simulink model "Elicottero2DOF_Sim"  (R2026a)
settings: Solver=VariableStepAuto  StopTime=20  FixedStep=0.0005
values from neighbouring files (symbols this model uses):
  M_0 = 46.5    [Elicottero2DOF_INIT.m]
  m_treshold = 3    [Elicottero2DOF_INIT.m]
  MAHALANOBIS = false    [Elicottero2DOF_INIT.m]
  Outlier_flag = 0    [Elicottero2DOF_INIT.m]
  P0 = diag([P_0_alpha P_0_alpha_dot P_0_beta P_0_beta_dot])    [Elicottero2DOF_INIT.m]
  q_0 = [alpha_0 beta_0]'    [Elicottero2DOF_INIT.m]
  q_dot_0 = [alpha_dot_0 beta_dot_0]'    [Elicottero2DOF_INIT.m]
  seme_rumore = 12345    [Elicottero2DOF_INIT.m]
  sigma_acc = 0.0137    [Elicottero2DOF_INIT.m]
  sigma_magn = 0.14    [Elicottero2DOF_INIT.m]
  st_acc = 0.00435    [Elicottero2DOF_INIT.m]
  st_magn = 0.005    [Elicottero2DOF_INIT.m]
  x_0 = [(deg2rad(10) + deg2rad(3)) 0.05 deg2rad(5) -0.05]'    [Elicottero2DOF_INIT.m]
undefined symbols (not defined in the file or in its folder): params
libraries: simulink x2
settings Model: Creator=giggi  LastModifiedBy=giggi

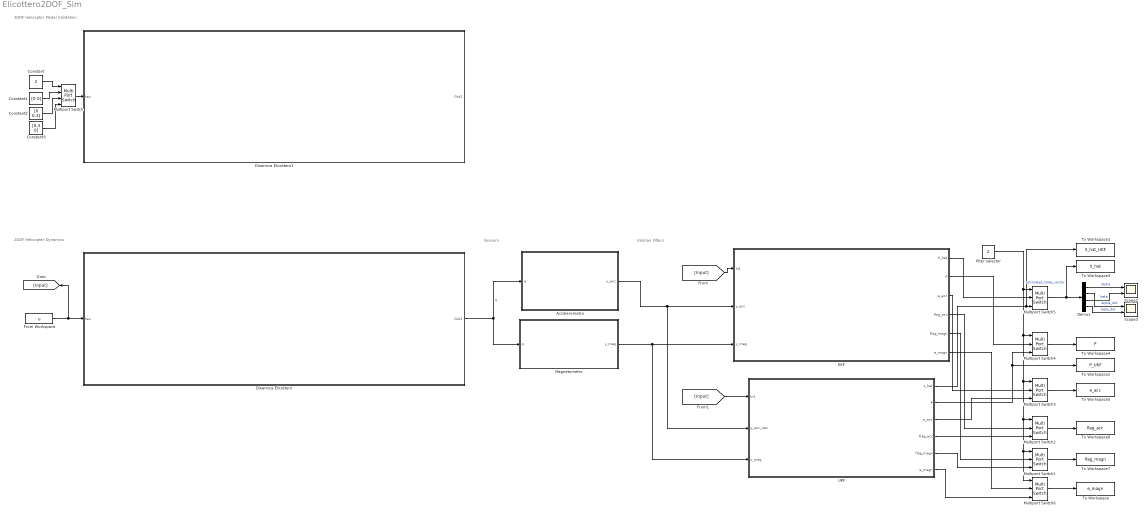
== system Elicottero2DOF_Sim ==
  note: Kalman FIlters
  note: 2DOF Helicopter Dynamics
  note: Sensors
  note: 2DOF Helicopter Model Validation
  Accelerometro : Subsystem
  Constant : Constant  Value=2
  Constant1 : Constant  Value=[0 0]
  Constant2 : Constant  Value=[0 0.3]
  Constant3 : Constant  Value=[0.3 0]
  Demux : Demux
  Dinamica Elicottero : Subsystem
  Dinamica Elicottero1 : Subsystem
  EKF : Subsystem
  From Workspace : FromWorkspace  VariableName=u  SampleTime=params.st
  Magnetometro : Subsystem
  Multiport Switch : MultiPortSwitch  SaturateOnIntegerOverflow=off  InputSameDT=off
  Multiport Switch{1..6} (6 alike) : MultiPortSwitch  Inputs=2  SaturateOnIntegerOverflow=off  InputSameDT=off
  Scope2 : Scope  NumInputPorts=2
      settings: ActiveDisplayYMinimum=-0.071075894197221115  ActiveDisplayYMaximum=0.60556663596837657  DataLoggingVariableName=ScopeData7
  Scope3 : Scope  NumInputPorts=2
      settings: ActiveDisplayYMinimum=-0.27957788580280007  ActiveDisplayYMaximum=0.23844227860003075  DataLoggingVariableName=ScopeData11
  To Workspace : ToWorkspace  VariableName=e_magn  SaveFormat=Timeseries  SampleTime=params.st
  To Workspace1 : ToWorkspace  VariableName=X_hat_UKF  SaveFormat=Timeseries  SampleTime=params.st
  To Workspace2 : ToWorkspace  VariableName=P_UKF  SaveFormat=Timeseries  SampleTime=params.st
  To Workspace3 : ToWorkspace  VariableName=X_hat  SaveFormat=Timeseries  SampleTime=params.st
  To Workspace4 : ToWorkspace  VariableName=P  SaveFormat=Timeseries  SampleTime=params.st
  To Workspace5 : ToWorkspace  VariableName=e_acc  SaveFormat=Timeseries  SampleTime=params.st
  To Workspace6 : ToWorkspace  VariableName=flag_acc  SaveFormat=Timeseries  SampleTime=params.st
  To Workspace7 : ToWorkspace  VariableName=flag_magn  SaveFormat=Timeseries  SampleTime=params.st
  UKF : Subsystem
  filter selector : Constant  Value=2
  wires:
  From Workspace/1 -> Dinamica Elicottero/1(tau), [Input]
  Dinamica Elicottero/1(Out1) -> Magnetometro/1(q), Accelerometro/1(q)  "q"
  [Input] -> EKF/1(In1)
  [Input] -> UKF/1(In1)
  Accelerometro/1(y_acc) -> UKF/2(y_acc_raw), EKF/2(y_acc)
  Magnetometro/1(y_mag) -> UKF/3(y_mag), EKF/3(y_mag)
  Constant/1 -> Multiport Switch/1
  Constant1/1 -> Multiport Switch/2
  Constant2/1 -> Multiport Switch/3
  Constant3/1 -> Multiport Switch/4
  Multiport Switch/1 -> Dinamica Elicottero1/1(tau)
  Demux/4 -> Scope3/2  "beta_dot"
  Demux/1 -> Scope2/1  "alpha"
  Demux/3 -> Scope2/2  "beta"
  Multiport Switch4/1 -> To Workspace4/1
  Demux/2 -> Scope3/1  "alpha_dot"
  Multiport Switch1/1 -> To Workspace7/1
  UKF/5(flag_magn) -> Multiport Switch1/3
  UKF/4(flag_acc) -> Multiport Switch2/3
  Multiport Switch2/1 -> To Workspace6/1
  UKF/3(e_acc) -> Multiport Switch3/3
  Multiport Switch3/1 -> To Workspace5/1
  Multiport Switch5/1 -> Demux/1, To Workspace3/1  "estimated_state_vector"
  UKF/2(P) -> Multiport Switch4/3, To Workspace2/1
  EKF/1(X_hat) -> Multiport Switch5/2
  UKF/1(x_hat) -> Multiport Switch5/3, To Workspace1/1
  EKF/2(P) -> Multiport Switch4/2
  EKF/3(e_acc) -> Multiport Switch3/2
  EKF/4(flag_acc) -> Multiport Switch2/2
  EKF/5(flag_magn) -> Multiport Switch1/2
  filter selector/1 -> Multiport Switch6/1, Multiport Switch1/1, Multiport Switch2/1, Multiport Switch3/1, Multiport Switch4/1, Multiport Switch5/1
  Multiport Switch6/1 -> To Workspace/1
  EKF/6(e_magn) -> Multiport Switch6/2
  UKF/6(e_magn) -> Multiport Switch6/3

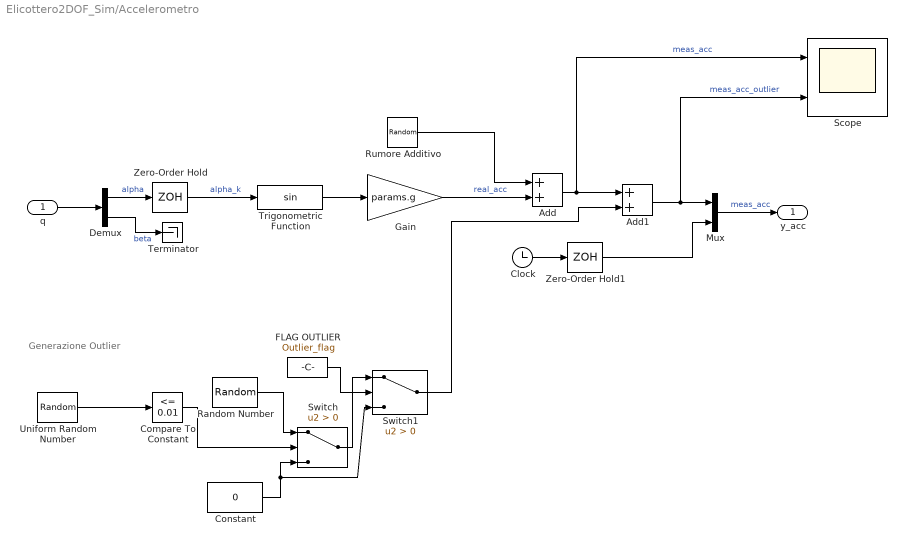
== system Elicottero2DOF_Sim/Accelerometro ==
  note: Generazione Outlier
  q : Inport
  Add : Sum
  Add1 : Sum
  Clock : Clock
  Compare To Constant : simulink/Logic and Bit Operations/Compare To Constant  relop=<=  const=0.01  OutDataTypeStr=boolean
  Constant : Constant  Value=0  SampleTime=st_acc
  Demux : Demux  Outputs=2
  FLAG OUTLIER : Constant  Value=Outlier_flag  SampleTime=st_acc
  Gain : Gain  Gain=params.g
  Mux : Mux  Inputs=2
  Random Number : RandomNumber  Variance=100  Seed=seme_rumore + 18  SampleTime=st_acc
  Rumore Additivo : RandomNumber  Variance=sigma_acc^2  Seed=seme_rumore  SampleTime=st_acc
  Scope : Scope  NumInputPorts=2
      settings: ActiveDisplayYMinimum=-1.7650304215432193  ActiveDisplayYMaximum=2.1182246618135347
  Switch : Switch  Criteria=u2 > Threshold  SaturateOnIntegerOverflow=off  InputSameDT=off
  Switch1 : Switch  Criteria=u2 > Threshold  SaturateOnIntegerOverflow=off  InputSameDT=off
  Terminator : Terminator
  Trigonometric Function : Trigonometry
  Uniform Random Number : UniformRandomNumber  Minimum=0  Seed=seme_rumore + 953  SampleTime=st_acc
  Zero-Order Hold : ZeroOrderHold  SampleTime=st_acc
  Zero-Order Hold1 : ZeroOrderHold  SampleTime=st_acc
  y_acc : Outport
  wires:
  q/1 -> Demux/1
  Demux/1 -> Zero-Order Hold/1  "alpha"
  Demux/2 -> Terminator/1  "beta"
  Trigonometric Function/1 -> Gain/1
  Gain/1 -> Add/2  "real_acc"
  Rumore Additivo/1 -> Add/1
  Add/1 -> Scope/1, Add1/1  "meas_acc"
  Zero-Order Hold/1 -> Trigonometric Function/1  "alpha_k"
  Mux/1 -> y_acc/1  "meas_acc"
  Clock/1 -> Zero-Order Hold1/1
  Zero-Order Hold1/1 -> Mux/2
  FLAG OUTLIER/1 -> Switch1/2
  Constant/1 -> Switch1/3, Switch/3
  Compare To Constant/1 -> Switch/2
  Random Number/1 -> Switch/1
  Switch/1 -> Switch1/1
  Switch1/1 -> Add1/2
  Uniform Random Number/1 -> Compare To Constant/1
  Add1/1 -> Scope/2, Mux/1  "meas_acc_outlier"

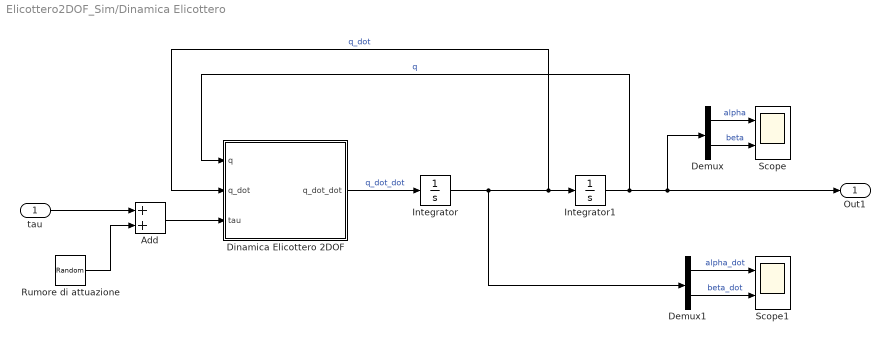
== system Elicottero2DOF_Sim/Dinamica Elicottero ==
  tau : Inport
  Add : Sum
  Demux : Demux  Outputs=2
  Demux1 : Demux  Outputs=2
  Dinamica Elicottero 2DOF : MATLAB Function  TreatAsAtomicUnit=on
  Integrator : Integrator  InitialCondition=q_dot_0
  Integrator1 : Integrator  InitialCondition=q_0
  Rumore di attuazione : RandomNumber  Mean=[0 0]  Variance=[params.sigma_F params.sigma_F].^2  Seed=seme_rumore + 15  SampleTime=params.st
  Scope : Scope  NumInputPorts=2
      settings: ActiveDisplayYMinimum=-0.1777950485917946  ActiveDisplayYMaximum=0.21368047784290267
  Scope1 : Scope  NumInputPorts=2
      settings: ActiveDisplayYMinimum=-0.28050979862132908  ActiveDisplayYMaximum=0.27285629021011787  DataLoggingVariableName=ScopeData4
  Out1 : Outport
  wires:
  Demux/1 -> Scope/1  "alpha"
  Integrator1/1 -> Out1/1, Demux/1, Dinamica Elicottero 2DOF/1(q)  "q"
  Dinamica Elicottero 2DOF/1(q_dot_dot) -> Integrator/1  "q_dot_dot"
  Demux/2 -> Scope/2  "beta"
  Demux1/1 -> Scope1/1  "alpha_dot"
  Demux1/2 -> Scope1/2  "beta_dot"
  Integrator/1 -> Demux1/1, Dinamica Elicottero 2DOF/2(q_dot), Integrator1/1  "q_dot"
  tau/1 -> Add/1
  Add/1 -> Dinamica Elicottero 2DOF/3(tau)
  Rumore di attuazione/1 -> Add/2

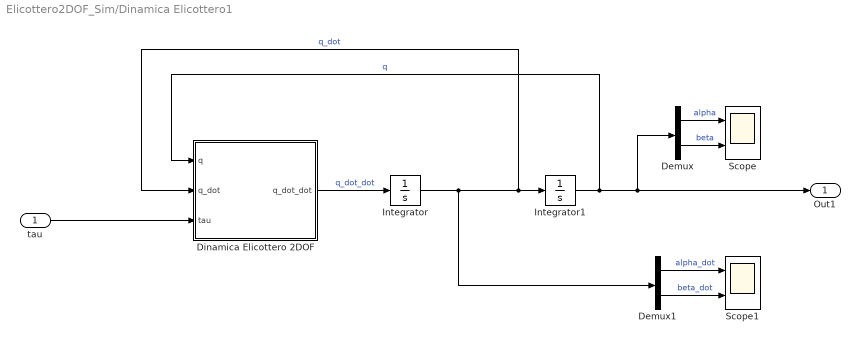
== system Elicottero2DOF_Sim/Dinamica Elicottero1 ==
  tau : Inport
  Demux : Demux  Outputs=2
  Demux1 : Demux  Outputs=2
  Dinamica Elicottero 2DOF : MATLAB Function  TreatAsAtomicUnit=on
  Integrator : Integrator  InitialCondition=q_dot_0
  Integrator1 : Integrator  InitialCondition=q_0
  Scope : Scope  NumInputPorts=2
      settings: ActiveDisplayYMinimum=-14.088875046539977  ActiveDisplayYMaximum=126.79987541885983
  Scope1 : Scope  NumInputPorts=2
      settings: ActiveDisplayYMinimum=-0.74875373653795674  ActiveDisplayYMaximum=6.7387836288416114  DataLoggingVariableName=ScopeData4
  Out1 : Outport
  wires:
  Demux/1 -> Scope/1  "alpha"
  Integrator1/1 -> Out1/1, Demux/1, Dinamica Elicottero 2DOF/1(q)  "q"
  Dinamica Elicottero 2DOF/1(q_dot_dot) -> Integrator/1  "q_dot_dot"
  Demux/2 -> Scope/2  "beta"
  Demux1/1 -> Scope1/1  "alpha_dot"
  Demux1/2 -> Scope1/2  "beta_dot"
  Integrator/1 -> Demux1/1, Dinamica Elicottero 2DOF/2(q_dot), Integrator1/1  "q_dot"
  tau/1 -> Dinamica Elicottero 2DOF/3(tau)

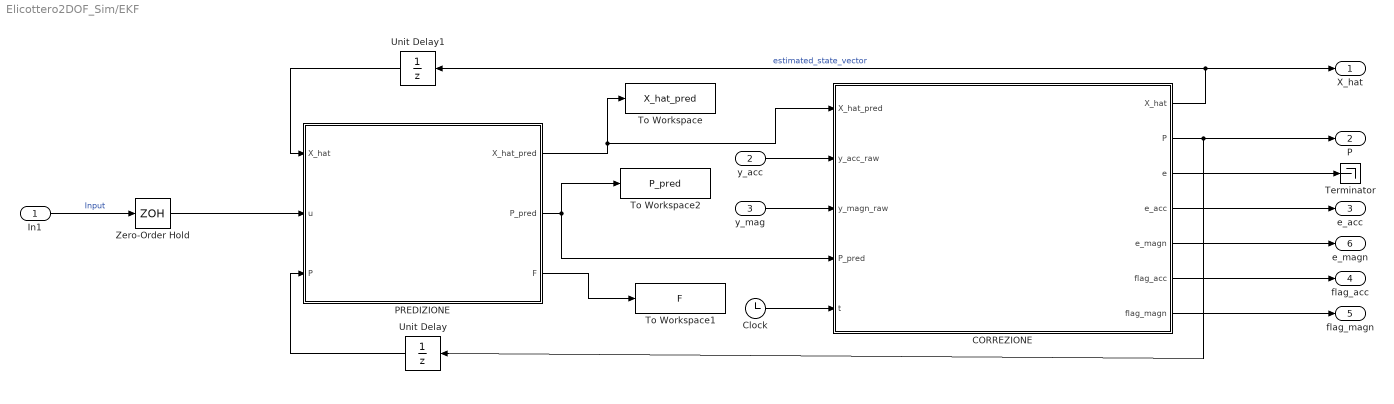
== system Elicottero2DOF_Sim/EKF ==
  In1 : Inport
  y_acc : Inport  Port=2
  y_mag : Inport  Port=3
  CORREZIONE : MATLAB Function  TreatAsAtomicUnit=on
  Clock : Clock
  PREDIZIONE : MATLAB Function  TreatAsAtomicUnit=on
  Terminator : Terminator
  To Workspace : ToWorkspace  VariableName=X_hat_pred  SaveFormat=Timeseries  SampleTime=params.st
  To Workspace1 : ToWorkspace  VariableName=F  SaveFormat=Timeseries  SampleTime=params.st
  To Workspace2 : ToWorkspace  VariableName=P_pred  SaveFormat=Timeseries  SampleTime=params.st
  Unit Delay : UnitDelay  InitialCondition=P0  SampleTime=params.st
  Unit Delay1 : UnitDelay  InitialCondition=x_0  SampleTime=params.st
  Zero-Order Hold : ZeroOrderHold  SampleTime=params.st
  X_hat : Outport
  P : Outport  Port=2
  e_acc : Outport  Port=3
  flag_acc : Outport  Port=4
  flag_magn : Outport  Port=5
  e_magn : Outport  Port=6
  wires:
  PREDIZIONE/2(P_pred) -> To Workspace2/1, CORREZIONE/4(P_pred)
  Zero-Order Hold/1 -> PREDIZIONE/2(u)
  In1/1 -> Zero-Order Hold/1  "Input"
  Unit Delay/1 -> PREDIZIONE/3(P)
  Unit Delay1/1 -> PREDIZIONE/1(X_hat)
  y_acc/1 -> CORREZIONE/2(y_acc_raw)
  y_mag/1 -> CORREZIONE/3(y_magn_raw)
  CORREZIONE/1(X_hat) -> X_hat/1, Unit Delay1/1  "estimated_state_vector"
  PREDIZIONE/1(X_hat_pred) -> To Workspace/1, CORREZIONE/1(X_hat_pred)
  CORREZIONE/2(P) -> Unit Delay/1, P/1
  Clock/1 -> CORREZIONE/5(t)
  PREDIZIONE/3(F) -> To Workspace1/1
  CORREZIONE/4(e_acc) -> e_acc/1
  CORREZIONE/6(flag_acc) -> flag_acc/1
  CORREZIONE/7(flag_magn) -> flag_magn/1
  CORREZIONE/3(e) -> Terminator/1
  CORREZIONE/5(e_magn) -> e_magn/1

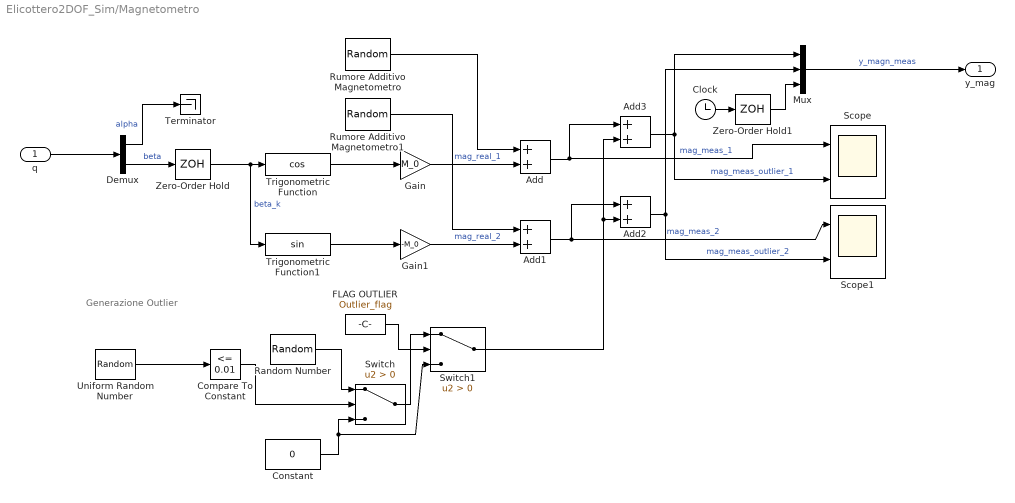
== system Elicottero2DOF_Sim/Magnetometro ==
  note: Generazione Outlier
  q : Inport
  Add{,1..3} (4 alike) : Sum
  Clock : Clock
  Compare To Constant : simulink/Logic and Bit Operations/Compare To Constant  relop=<=  const=0.01  OutDataTypeStr=boolean
  Constant : Constant  Value=0  SampleTime=st_magn
  Demux : Demux  Outputs=2
  FLAG OUTLIER : Constant  Value=Outlier_flag  SampleTime=st_magn
  Gain : Gain  Gain=M_0
  Gain1 : Gain  Gain=-M_0
  Mux : Mux  Inputs=3
  Random Number : RandomNumber  Variance=100  Seed=seme_rumore + 43  SampleTime=st_magn
  Rumore Additivo Magnetometro : RandomNumber  Variance=sigma_magn^2  Seed=seme_rumore + 1  SampleTime=st_magn
  Rumore Additivo Magnetometro1 : RandomNumber  Variance=sigma_magn^2  Seed=seme_rumore + 300  SampleTime=st_magn
  Scope : Scope  NumInputPorts=2
      settings: ActiveDisplayYMinimum=45.876225966404974  ActiveDisplayYMaximum=47.084900080547662  DataLoggingVariableName=ScopeData2
  Scope1 : Scope  NumInputPorts=2
      settings: ActiveDisplayYMinimum=-0.62118665847594379  ActiveDisplayYMaximum=0.61456044976709734  DataLoggingVariableName=ScopeData3
  Switch : Switch  Criteria=u2 > Threshold  SaturateOnIntegerOverflow=off  InputSameDT=off
  Switch1 : Switch  Criteria=u2 > Threshold  SaturateOnIntegerOverflow=off  InputSameDT=off
  Terminator : Terminator
  Trigonometric Function : Trigonometry  Operator=cos
  Trigonometric Function1 : Trigonometry
  Uniform Random Number : UniformRandomNumber  Minimum=0  Seed=seme_rumore + 921  SampleTime=st_magn
  Zero-Order Hold : ZeroOrderHold  SampleTime=st_magn
  Zero-Order Hold1 : ZeroOrderHold  SampleTime=st_magn
  y_mag : Outport
  wires:
  q/1 -> Demux/1
  Demux/2 -> Zero-Order Hold/1  "beta"
  Demux/1 -> Terminator/1  "alpha"
  Trigonometric Function/1 -> Gain/1
  Trigonometric Function1/1 -> Gain1/1
  Gain/1 -> Add/2  "mag_real_1"
  Rumore Additivo Magnetometro/1 -> Add/1
  Gain1/1 -> Add1/2  "mag_real_2"
  Zero-Order Hold/1 -> Trigonometric Function1/1, Trigonometric Function/1  "beta_k"
  Mux/1 -> y_mag/1  "y_magn_meas"
  Clock/1 -> Zero-Order Hold1/1
  Zero-Order Hold1/1 -> Mux/3
  Uniform Random Number/1 -> Compare To Constant/1
  Random Number/1 -> Switch/1
  Compare To Constant/1 -> Switch/2
  Constant/1 -> Switch1/3, Switch/3
  FLAG OUTLIER/1 -> Switch1/2
  Switch/1 -> Switch1/1
  Add/1 -> Scope/1, Add3/1  "mag_meas_1"
  Rumore Additivo Magnetometro1/1 -> Add1/1
  Add2/1 -> Scope1/2, Mux/2  "mag_meas_outlier_2"
  Add1/1 -> Scope1/1, Add2/1  "mag_meas_2"
  Switch1/1 -> Add2/2, Add3/2
  Add3/1 -> Scope/2, Mux/1  "mag_meas_outlier_1"

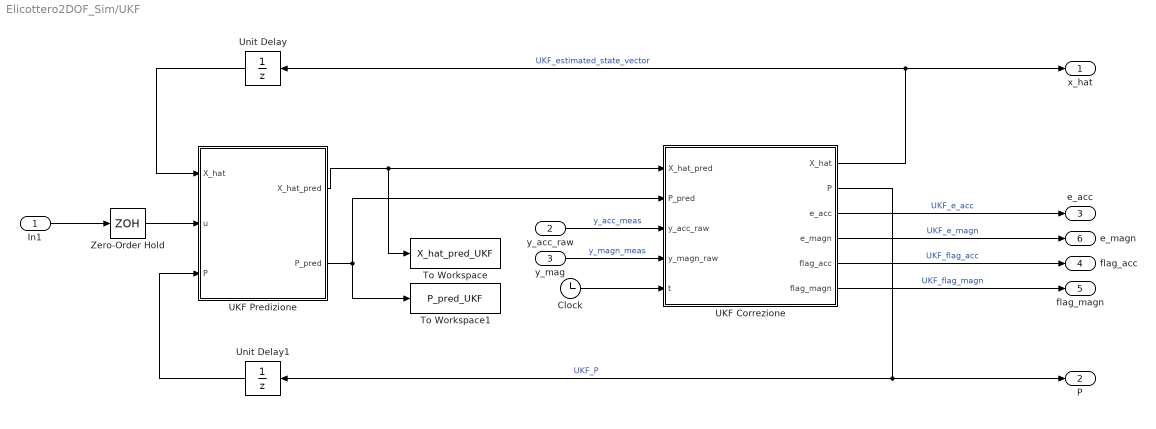
== system Elicottero2DOF_Sim/UKF ==
  In1 : Inport
  y_acc_raw : Inport  Port=2
  y_mag : Inport  Port=3
  Clock : Clock
  To Workspace : ToWorkspace  VariableName=X_hat_pred_UKF  SaveFormat=Timeseries  SampleTime=params.st
  To Workspace1 : ToWorkspace  VariableName=P_pred_UKF  SaveFormat=Timeseries  SampleTime=params.st
  UKF Correzione : MATLAB Function  TreatAsAtomicUnit=on
  UKF Predizione : MATLAB Function  TreatAsAtomicUnit=on
  Unit Delay : UnitDelay  InitialCondition=x_0  SampleTime=params.st
  Unit Delay1 : UnitDelay  InitialCondition=P0  SampleTime=params.st
  Zero-Order Hold : ZeroOrderHold  SampleTime=params.st
  x_hat : Outport
  P : Outport  Port=2
  e_acc : Outport  Port=3
  flag_acc : Outport  Port=4
  flag_magn : Outport  Port=5
  e_magn : Outport  Port=6
  wires:
  Unit Delay/1 -> UKF Predizione/1(X_hat)
  Unit Delay1/1 -> UKF Predizione/3(P)
  In1/1 -> Zero-Order Hold/1
  Zero-Order Hold/1 -> UKF Predizione/2(u)
  y_acc_raw/1 -> UKF Correzione/3(y_acc_raw)  "y_acc_meas"
  y_mag/1 -> UKF Correzione/4(y_magn_raw)  "y_magn_meas"
  UKF Predizione/1(X_hat_pred) -> To Workspace/1, UKF Correzione/1(X_hat_pred)
  UKF Predizione/2(P_pred) -> To Workspace1/1, UKF Correzione/2(P_pred)
  UKF Correzione/1(X_hat) -> x_hat/1, Unit Delay/1  "UKF_estimated_state_vector"
  UKF Correzione/2(P) -> P/1, Unit Delay1/1  "UKF_P"
  UKF Correzione/3(e_acc) -> e_acc/1  "UKF_e_acc"
  Clock/1 -> UKF Correzione/5(t)
  UKF Correzione/6(flag_magn) -> flag_magn/1  "UKF_flag_magn"
  UKF Correzione/5(flag_acc) -> flag_acc/1  "UKF_flag_acc"
  UKF Correzione/4(e_magn) -> e_magn/1  "UKF_e_magn"

== matlab function Elicottero2DOF_Sim/Dinamica Elicottero1/Dinamica Elicottero 2DOF ==
  data: q input; q_dot input; tau input; q_dot_dot output; params parameter
function q_dot_dot = fcn(q, q_dot, tau, params)

alpha = q(1);
alpha_dot = q_dot(1);
beta = q(2);
beta_dot = q_dot(2);

% Costruzione Momento di Inerzia di Yaw (Variabile con angolo di pitch)
J_beta = params.J_y * sin(alpha)^2 + (params.J_z + params.m * params.l^2) * cos(alpha)^2 + params.I_b;

% Matrice di Inerzia
M = [params.J_alpha 0; 0 J_beta];

% Vettore dei termini non lineari (raccoglie attriti viscosi e forza di gravità)
n = [params.c_alpha * alpha_dot + params.m * params.g * params.l * sin(alpha); params.c_beta * beta_dot];

% Vettore delle Forze / Coppie generalizzate
B = [params.l * cos(beta), params.epsilon_p * params.l * sin(beta); params.epsilon_y * params.l * sin(alpha), params.l * cos(alpha)];

% Dinamica Inversa
q_dot_dot = M \ (B * tau - n);

== matlab function Elicottero2DOF_Sim/EKF/PREDIZIONE ==
  data: X_hat input; u input; P input; X_hat_pred output; P_pred output; params parameter; F output
function [X_hat_pred, P_pred, F] = Predizione(X_hat, u, P, params)
    % PREDIZIONE EKF - Modello con Rumore di Attuazione sui Motori
    
    %% 1. Lettura dello Stato e Ingressi
    alpha     = X_hat(1);
    alpha_dot = X_hat(2);
    beta      = X_hat(3);
    beta_dot  = X_hat(4);
    
    F1 = u(1);
    F2 = u(2);
    
    %% 2. Estrazione Parametri Fisici
    m  = params.m;       l  = params.l;       g  = params.g;
    Ja = params.J_alpha; Jy = params.J_y;     Jz = params.J_z;
    Ib = params.I_b;     ca = params.c_alpha; cb = params.c_beta;
    ep = params.epsilon_p;   ey = params.epsilon_y;   
    dt = params.st;
    
    %% 3. Matrice di Covarianza del Rumore di Processo (Q)
    % Q è 2x2. Contiene la varianza del rumore dei motori EMAX MT2204
    % param.sigma_F = 0.05 [Newton]
    Q = [params.sigma_F^2, 0;
         0,               params.sigma_F^2];

    %% 4. MODELLO DINAMICO NON LINEARE
    J_beta = Jy * sin(alpha)^2 + (Jz + m*l^2) * cos(alpha)^2 + Ib;
    
    alpha_ddot = (-ca * alpha_dot - m * g * l * sin(alpha) + ...
                   l * F1 * cos(beta) + ep * l * F2 * sin(beta)) / Ja;
                   
    beta_ddot  = (-cb * beta_dot + l * F2 * cos(alpha) + ...
                   ey * l * F1 * sin(alpha)) / J_beta;

    %% 5. PREDIZIONE DELLO STATO (Eulero)
    X_hat_pred = [alpha     + dt * alpha_dot;
                  alpha_dot + dt * alpha_ddot;
                  beta      + dt * beta_dot;
                  beta_dot  + dt * beta_ddot];

    %% 6. CALCOLO JACOBIANA DI PROCESSO (A) -> F = I + A*dt
    % Derivate per la riga 2 (alpha_ddot)
    A21 = (-m * g * l * cos(alpha)) / Ja;
    A22 = -ca / Ja;
    A23 = (-l * F1 * sin(beta) + ep * l * F2 * cos(beta)) / Ja;
    A24 = 0;
    
    % Derivate per la riga 4 (beta_ddot)
    N = -cb * beta_dot + l * F2 * cos(alpha) + ey * l * F1 * sin(alpha);
    D_den = J_beta;
    dN_dalpha = -l * F2 * sin(alpha) + ey * l * F1 * cos(alpha);
    dD_dalpha = 2 * Jy * sin(alpha) * cos(alpha) - 2 * (Jz + m*l^2) * cos(alpha) * sin(alpha);
    
    A41 = (D_den * dN_dalpha - N * dD_dalpha) / (D_den^2);
    A42 = 0;
    A43 = 0;
    A44 = -cb / D_den;
    
    % Assemblaggio e discretizzazione
    A = [  0,   1,   0,   0;
         A21, A22, A23, A24;
           0,   0,   0,   1;
         A41, A42, A43, A44];
         
    F = eye(4) + A * dt;
    
    %% 7. CALCOLO JACOBIANA DEI DISTURBI (D)
    % Rappresenta l'impatto di 1 Newton di errore del motore sulle accelerazioni.
    % La matrice è 4x2 perché mappa 2 rumori su 4 stati.
    
    d_alpha_ddot_w1 = (l * cos(beta)) / Ja;
    d_alpha_ddot_w2 = (ep * l * sin(beta)) / Ja;
    
    d_beta_ddot_w1  = (ey * l * sin(alpha)) / J_beta;
    d_beta_ddot_w2  = (l * cos(alpha)) / J_beta;
    
    D = [0,                         0;
         d_alpha_ddot_w1 * dt,      d_alpha_ddot_w2 * dt;
         0,                         0;
         d_beta_ddot_w1 * dt,       d_beta_ddot_w2 * dt];
         
    %% 8. PREDIZIONE DELLA COVARIANZA
    % Diffusione dell'incertezza dei motori negli stati tramite la matrice D
    P_pred = F * P * F' + D * Q * D';
    
end

== matlab function Elicottero2DOF_Sim/Dinamica Elicottero/Dinamica Elicottero 2DOF ==
  data: q input; q_dot input; tau input; q_dot_dot output; params parameter
function q_dot_dot = fcn(q, q_dot, tau, params)

alpha = q(1);
alpha_dot = q_dot(1);
beta = q(2);
beta_dot = q_dot(2);

% Costruzione Momento di Inerzia di Yaw (Variabile con angolo di pitch)
J_beta = params.J_y * sin(alpha)^2 + (params.J_z + params.m * params.l^2) * cos(alpha)^2 + params.I_b;

% Matrice di Inerzia
M = [params.J_alpha 0; 0 J_beta];

% Vettore dei termini non lineari (raccoglie attriti viscosi e forza di gravità)
n = [params.c_alpha * alpha_dot + params.m * params.g * params.l * sin(alpha); params.c_beta * beta_dot];

% Vettore delle Forze / Coppie generalizzate
B = [params.l * cos(beta), params.epsilon_p * params.l * sin(beta); params.epsilon_y * params.l * sin(alpha), params.l * cos(alpha)];

% Dinamica Inversa
q_dot_dot = M \ (B * tau - n);

== matlab function Elicottero2DOF_Sim/EKF/CORREZIONE ==
  data: X_hat_pred input; y_acc_raw input; y_magn_raw input; X_hat output; P_pred input; P output; params parameter; t input; MAHALANOBIS parameter; M_0 parameter; e output; e_acc output; e_magn output; m_treshold parameter; flag_acc output; flag_magn output
function [X_hat, P, e, e_acc,e_magn, flag_acc,flag_magn] = Correzione(X_hat_pred, y_acc_raw, y_magn_raw, P_pred, params, t, MAHALANOBIS, M_0, m_treshold)
    % FUNZIONE DI CORREZIONE EKF 
    % Modello di osservazione: 
    % y_acc = gsin(alpha_k) + v_alpha_k
    % y_magn = [M_0*cos*(beta_k),-M_0*sin(beta_k)] + [v_beta_k, v_beta_k]

    g = params.g;
    dt = params.st;

    % Inizializzazione
    X_hat = X_hat_pred;
    P = P_pred;
    
    % Input (x_k|k-1)
    alpha = X_hat_pred(1); 
    beta = X_hat_pred(3);

    % Uscite Sensori
    t_acc = y_acc_raw(2);
    t_magn = y_magn_raw(3);
    y_acc = y_acc_raw(1);
    y_magn = y_magn_raw(1:2);

      
    % Covarianze errore di misura
    R = diag([params.R_acc, params.R_magn, params.R_magn]);
    
    % Matrice M = dh_k/dv_k  valutata in x_k|k-1
    M = eye(3);

    % Matrice H = dh_k/x_k valutata in x_k|k-1
    H = [g*cos(alpha), 0, 0, 0; ...
        0, 0, -M_0*sin(beta), 0; ...
        0, 0, -M_0*cos(beta), 0];

    % Innovazione
    e = [y_acc; y_magn] - [g*sin(alpha); M_0*cos(beta);-M_0*sin(beta)];

    % Calcolo delle singole distanze di mahalanobis
    H_acc = H(1, :);
    e_acc = e(1);
    M_acc = M(1, 1);
    R_acc = R(1, 1);
    S_acc = H_acc * P_pred * H_acc' + M_acc * R_acc * M_acc';
    mahalanobis_acc = sqrt(e_acc' / S_acc * e_acc);

    H_magn = H(2:3, :);
    e_magn = e(2:3);
    M_magn = M(2:3, 2:3);
    R_magn = R(2:3, 2:3);
    S_magn = H_magn * P_pred * H_magn' + M_magn * R_magn * M_magn';
    mahalanobis_magn = sqrt(e_magn' / S_magn * e_magn);

    % Verifica della disponibilità delle misure
    if MAHALANOBIS
        flag_acc = (mahalanobis_acc <= m_treshold) && (t_acc <= t) && (t - dt < t_acc);
        flag_magn = (mahalanobis_magn <= m_treshold) && (t_magn <= t) && (t - dt < t_magn);
    else
        flag_acc =  (t_acc <= t) && (t - dt < t_acc);
        flag_magn = (t_magn <= t) && (t - dt < t_magn);
    end

    % Costruzione delle matrici in base alle misure valide
    % Entrambe le misure valide
    if flag_acc && flag_magn
        H_curr = H;
        e_curr = e;
        M_curr = M;
        R_curr = R;

    elseif flag_acc     % Solo misura accelerometro disponibile
        H_curr = H_acc;
        e_curr = e_acc;
        M_curr = M_acc;
        R_curr = R_acc;

    elseif flag_magn    % Solo misura magnetometro disponibile
        H_curr = H_magn;
        e_curr = e_magn;
        M_curr = M_magn;
        R_curr = R_magn;

    else                % Nessuna misura disponibile
        return;
    end

    % Covarianza dell'innovazione
    S = H_curr * P_pred * H_curr' + M_curr * R_curr * M_curr';

    % Guadagno di Correzione
    L = P_pred * H_curr' / S;
    
    % Aggiornamento stato e covarianza
    X_hat = X_hat_pred + L * e_curr;
    % Forma di Joseph
    P = (eye(4) - L * H_curr) * P_pred * (eye(4) - L * H_curr)' + L * R_curr * L';

end

== matlab function Elicottero2DOF_Sim/UKF/UKF Predizione ==
  data: X_hat input; u input; params parameter; X_hat_pred output; P input; P_pred output
function [X_hat_pred, P_pred] = UKF_Predizione(X_hat,u, params, P)

lambda = params.lambda;
n = params.n;

n_state = params.n_state;

% Estrazione parametri

m = params.m;   J_a = params.J_alpha;   l = params.l;
g = params.g;   c_a = params.c_alpha;   c_b = params.c_beta;
e_p = params.epsilon_p;     e_y = params.epsilon_y;

F_1 = u(1);
F_2 = u(2);

% Inizializzazione vettore sigma_points
sigma_points = zeros(n, 2*n + 1);

Q = diag([params.sigma_F^2, params.sigma_F^2]);

P_a = blkdiag(P, Q);

% Definizione stato aumentato
X_a = [X_hat; zeros(params.n_input, 1)];

% 1. Decomposizione ai Valori Singolari (SVD)
[U, S, ~] = svd(P_a); 

% 2. Protezione Numerica Assoluta: 
% Trasforma eventuali autovalori microscopici negativi in zero
S_positiva = max(S, 0); 

% 3. Calcolo della Radice di Matrice
GAMMA = U * sqrt(S_positiva);

% Estrazione Sigma-points(da -n ad n)
for i =-n:n
    idx = i + n + 1;
    if i == 0      
        sigma_points(:, idx) = X_a;       % Sigma-point centrale
    elseif i > 0
        sigma_points(:, idx) = X_a + sqrt(n + lambda) * GAMMA(:, i);
    elseif i < 0
        sigma_points(:, idx) = X_a - sqrt(n + lambda) * GAMMA(:, abs(i));
    end
end


%--------------------------------------------------------------------------
% PROPAGAZIONE SIGMA-POINTS
%--------------------------------------------------------------------------

sigma_points_pred = zeros(n_state, 2*n + 1);

dt = params.st;

for i = 1:(2*n + 1)

    % Estrazione Stato
    alpha = sigma_points(1, i);
    alpha_dot = sigma_points(2, i);
    beta = sigma_points(3, i);
    beta_dot = sigma_points(4, i);

    % Estrazione rumore di attuazione
    w_1 = sigma_points(5, i);
    w_2 = sigma_points(6, i);

    F_1_noise = F_1 + w_1;
    F_2_noise = F_2 + w_2;


    % Dinamica del sistema
    J_beta = params.J_y * sin(alpha)^2 + (params.J_z + params.m * params.l^2) * cos(alpha)^2 + params.I_b;

    alpha_dot_dot = 1/J_a * (-c_a * alpha_dot - m* g * l * sin(alpha) + l * F_1_noise * cos(beta) + e_p * l * F_2_noise * sin(beta));
    beta_dot_dot = 1/J_beta * (-c_b * beta_dot + l * F_2_noise * cos(alpha) + e_y * l * F_1_noise * sin(alpha));
    

    % Eulero:
    sigma_points_pred(1, i) = alpha + dt * alpha_dot;
    sigma_points_pred(2, i) = alpha_dot + dt * alpha_dot_dot;
    sigma_points_pred(3, i) = beta + dt * beta_dot;
    sigma_points_pred(4, i) = beta_dot + dt * beta_dot_dot;

end



% Predizione
X_hat_pred = zeros(4, 1);
for i = 1:(2*n + 1)
    X_hat_pred = X_hat_pred + params.Wm(i) * sigma_points_pred(:, i);
end

P_pred = zeros(4, 4);

for i = 1:(2*n + 1)
    P_pred = P_pred + params.Wc(i) * (sigma_points_pred(:, i) - X_hat_pred) * (sigma_points_pred(:, i) - X_hat_pred)';
end

end

== matlab function Elicottero2DOF_Sim/UKF/UKF Correzione ==
  data: X_hat_pred input; X_hat output; P output; e_acc output; e_magn output; flag_acc output; P_pred input; y_acc_raw input; y_magn_raw input; params parameter; M_0 parameter; MAHALANOBIS parameter; m_treshold parameter; t input; flag_magn output
function [X_hat, P, e_acc,e_magn,flag_acc, flag_magn] = UKF_Correzione(X_hat_pred, P_pred, y_acc_raw, y_magn_raw, params, M_0, MAHALANOBIS, m_treshold, t)
% CORREZIONE UKF, conviene sfruttare il fatto che il rumore di misura è
% additivo (in questo caso non avrò lo stato aumentato con i rumori di
% misura)

n_state = params.n_state;
lambda = params.lambda_c;
g = params.g;
dt = params.st;

% Pre-allocazione (se nessuna misura è disponibile, rimango con la
% stima predetta)
P = P_pred;
X_hat = X_hat_pred;

% Uscite sensori
y_acc = y_acc_raw(1);
t_acc = y_acc_raw(2);

y_magn = y_magn_raw(1:2);
t_magn = y_magn_raw(3);

% Inizializzazione vettore sigma_points
sigma_points = zeros(n_state, 2*n_state + 1);

% 1. Decomposizione ai Valori Singolari (SVD)
[U, S, ~] = svd((P_pred + P_pred')/2); 

% 2. Protezione Numerica Assoluta: 
% Trasforma eventuali autovalori microscopici negativi in zero
S_positiva = max(S, 0); 

% 3. Calcolo della Radice di Matrice
GAMMA = U * sqrt(S_positiva);

% Estrazione Sigma-points(da -n_state ad n_state)
for i =-n_state:n_state
    idx = i + n_state + 1;
    if i == 0      
        sigma_points(:, idx) = X_hat_pred;       % Sigma-point centrale
    elseif i > 0
        sigma_points(:, idx) = X_hat_pred + sqrt(n_state + lambda) * GAMMA(:, i);
    elseif i < 0
        sigma_points(:, idx) = X_hat_pred - sqrt(n_state + lambda) * GAMMA(:, abs(i));
    end
end

%--------------------------------------------------------------------------
% PROPAGAZIONE ATTRAVERSO I SENSORI (TRASFORMATA UNSCENTED)
%--------------------------------------------------------------------------
Y_points = zeros(3, 2*n_state + 1);
for i = 1:(2*n_state +1)

    alpha = sigma_points(1, i);
    beta = sigma_points(3, i);

    % Modello di osservazione
    Y_points(1, i) = g * sin(alpha);
    Y_points(2, i) = M_0 * cos(beta);
    Y_points(3, i) = -M_0 * sin(beta);

end

% Media
y_hat = zeros(3, 1);
for i = 1:(2*n_state + 1)
    y_hat = y_hat + params.Wm_c(i) * Y_points(:, i);
end

% Covarianza
P_yy = zeros(3, 3);
P_xy = zeros(n_state, 3);
for i = 1:(2*n_state + 1)
    P_yy = P_yy + params.Wc_c(i) * ((Y_points(:, i) - y_hat) * (Y_points(:, i) - y_hat)');
    P_xy = P_xy + params.Wc_c(i) * ((sigma_points(:, i) - X_hat_pred) * (Y_points(:, i) - y_hat)');
end


%--------------------------------------------------------------------------
% Calcolo delle distanze di mahalanobis per i singoli sensori
%--------------------------------------------------------------------------

e = [y_acc; y_magn] - y_hat;

R = diag([params.R_acc, params.R_magn, params.R_magn]);

% Accelerometro
e_acc = e(1);
R_acc = R(1, 1);
S_acc = P_yy(1, 1) + R_acc;     % Sfrutto rumore additivo
mahalanobis_acc = sqrt(e_acc' / S_acc * e_acc);

% Magnetometro
e_magn = e(2:3);
R_magn = R(2:3, 2:3);
S_magn = P_yy(2:3, 2:3) + R_magn;
mahalanobis_magn = sqrt(e_magn' / S_magn * e_magn);

% Verifica della disponibilità delle misure
if MAHALANOBIS
    flag_acc = (mahalanobis_acc <= m_treshold) && (t_acc <= t) && (t - dt < t_acc);
    flag_magn = (mahalanobis_magn <= m_treshold) && (t_magn <= t) && (t - dt < t_magn);
else
    flag_acc =  (t_acc <= t) && (t - dt < t_acc);
    flag_magn = (t_magn <= t) && (t - dt < t_magn);
end


% Costruzione delle matrici in base alle misure valide
% Entrambe le misure valide
if flag_acc && flag_magn

    e_curr = e;
    S_curr = P_yy + R;
    P_xy_curr = P_xy;
    
elseif flag_acc     % Solo misura accelerometro disponibile
    e_curr = e_acc;
    S_curr = S_acc;
    P_xy_curr = P_xy(:, 1);

elseif flag_magn    % Solo misura magnetometro disponibile
    e_curr = e_magn;
    S_curr = S_magn;
    P_xy_curr = P_xy(:, 2:3);

else                % Nessuna misura disponibile
    return;
end

% CORREZIONE
% Guadagno di correzione
L = P_xy_curr / S_curr;

% x_k|k
X_hat = X_hat_pred + L * e_curr;

% P_k|k 
P = P_pred - L * S_curr * L';
